simulink model "euler_equation_dave"  (R2021b)
settings: Solver=VariableStepAuto  StartTime=0.0  StopTime=30  MaxStep=0.01  RelTol=1e-3
values from neighbouring files (symbols this model uses):
  a = 2.4501e+4    (= 24501)    [heliocentric_plot.m]    (also in parameters_euler_equations_dave.m = 10500)
  e = 0.6665    [heliocentric_plot.m]    (also in parameters_euler_equations_dave.m = 0)
  Euler0131 = [0 pi/4 0]'    [parameters_euler_equations_dave.m]
  Euler0312 = [pi/4, 0, 0]'    [parameters_euler_equations_dave.m]
  h_versor = h ./ (h_norm)    [parameters_euler_equations_dave.m]
  I = [I_x_body, I_y_body, I_z_body]    [parameters_euler_equations_dave.m]
  i_0 = 0    [parameters_euler_equations_dave.m]
  J = diag (I)    [parameters_euler_equations_dave.m]
  J_inv = inv(J)    [parameters_euler_equations_dave.m]
  Mat_g = g .* S * 1e-09    [ghnorm.m]
  Mat_gsv = gsv .* S*  1e-09    [ghnorm.m]
  Mat_h = h .* S * 1e-09    [ghnorm.m]
  Mat_hsv = hsv .* S*  1e-09    [ghnorm.m]
  muP = astroConstants(13)    [parameters_euler_equations_dave.m]
  n = mat(:, 1)    [ghnorm.m]    (also in parameters_euler_equations_dave.m = 2*pi/T)
  N = max(mat (:, 2))    [ghnorm.m]    (also in parameters_euler_equations_dave.m = [n1 n2 n3 n4 n5 n6])
  n_sun = 2*pi/(365*24*3600)    (= 1.99238499086e-07)    [parameters_euler_equations_dave.m]    (also in srp.m = 1.99102127766e-07)
  R_sun = 149600000    [parameters_euler_equations_dave.m]
  Sat_dim = [a_body b_body c_body]    [parameters_euler_equations_dave.m]
  star1_in = [Sx(1); Sy(1); Sz(1)]    [parameters_euler_equations_dave.m]    (also in stars.m)
  star2_in = [Sx(2); Sy(2); Sz(2)]    [parameters_euler_equations_dave.m]    (also in stars.m)
  star3_in = [Sx(3); Sy(3); Sz(3)]    [parameters_euler_equations_dave.m]    (also in stars.m)
  theta_g0 = 0    [parameters_euler_equations_dave.m]
  true_anomaly0 = 0    [parameters_euler_equations_dave.m]
  Ts = 0.1    [parameters_euler_equations_dave.m]
  w0 = [wx, wy, wz]    [parameters_euler_equations_dave.m]
undefined symbols (not defined in the file or in its folder): A_SB, g_mat, h_mat, init_mjd2000, magnetic_torque, r0, t0, v0, vec_norm, we
libraries: sharedutil x13, vrlib x8, simulink_extras x6, sharedtransform x5, matrix_library x3, aerolibconvert2 x2, euler x1
(part 2 of 2)

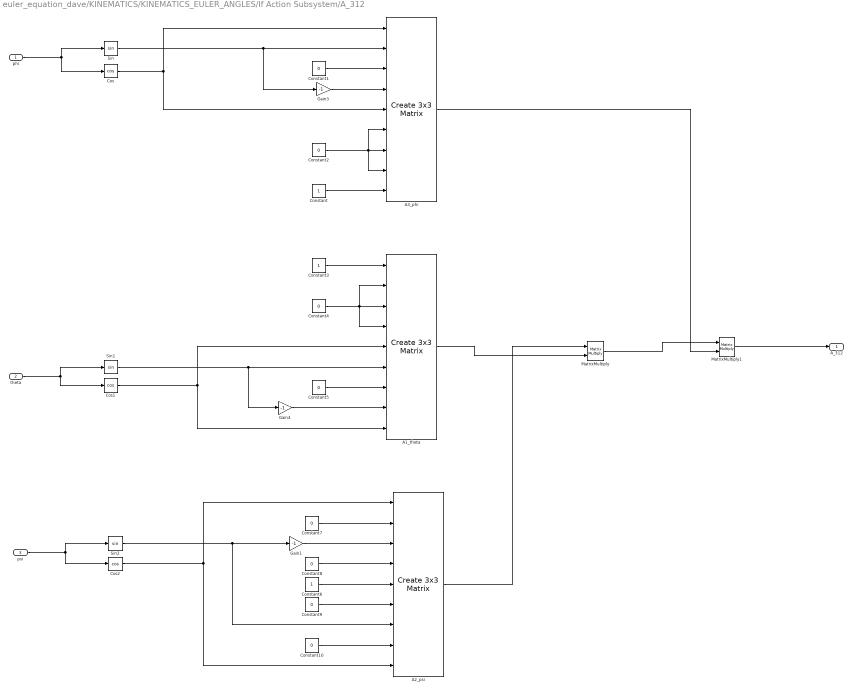
== system euler_equation_dave/KINEMATICS/KINEMATICS_EULER_ANGLES/If Action Subsystem/A_312 ==
  phi : Inport
  theta : Inport  Port=2
  psi : Inport  Port=3
  A1_theta : sharedutil/Create 3x3 Matrix  aMode=aMode
      settings: SourceProductBaseCode=AE,PW,DR,MT,UV,VE
  A2_psi : sharedutil/Create 3x3 Matrix  aMode=aMode
      settings: SourceProductBaseCode=AE,PW,DR,MT,UV,VE
  A3_phi : sharedutil/Create 3x3 Matrix  aMode=aMode
      settings: SourceProductBaseCode=AE,PW,DR,MT,UV,VE
  Constant : Constant
  Constant{1..2,4..5,7..10} (8 alike) : Constant  Value=0
  Constant3 : Constant
  Constant6 : Constant
  Cos : Trigonometry  Operator=cos
  Cos1 : Trigonometry  Operator=cos
  Cos2 : Trigonometry  Operator=cos
  Gain1 : Gain  Gain=-1
  Gain3 : Gain  Gain=-1
  Gain4 : Gain  Gain=-1
  MatrixMultiply : Product  Multiplication=Matrix(*)
  MatrixMultiply1 : Product  Multiplication=Matrix(*)
  Sin : Trigonometry
  Sin1 : Trigonometry
  Sin2 : Trigonometry
  A_312 : Outport
  wires:
  phi/1 -> Sin/1, Cos/1
  theta/1 -> Sin1/1, Cos1/1
  psi/1 -> Sin2/1, Cos2/1
  Cos/1 -> A3_phi/5, A3_phi/1
  Sin/1 -> A3_phi/2, Gain3/1
  Constant/1 -> A3_phi/9
  Constant1/1 -> A3_phi/3
  Constant2/1 -> A3_phi/8, A3_phi/6, A3_phi/7
  Constant3/1 -> A1_theta/1
  Constant4/1 -> A1_theta/4, A1_theta/3, A1_theta/2
  Cos1/1 -> A1_theta/5, A1_theta/9
  Constant5/1 -> A1_theta/7
  Cos2/1 -> A2_psi/9, A2_psi/1
  Constant7/1 -> A2_psi/2
  Constant9/1 -> A2_psi/6
  Constant8/1 -> A2_psi/4
  Constant6/1 -> A2_psi/5
  Sin2/1 -> A2_psi/7, Gain1/1
  Constant10/1 -> A2_psi/8
  A2_psi/1 -> MatrixMultiply/1
  A1_theta/1 -> MatrixMultiply/2
  MatrixMultiply/1 -> MatrixMultiply1/1
  A3_phi/1 -> MatrixMultiply1/2
  MatrixMultiply1/1 -> A_312/1
  Sin1/1 -> A1_theta/6, Gain4/1
  Gain3/1 -> A3_phi/4
  Gain4/1 -> A1_theta/8
  Gain1/1 -> A2_psi/3

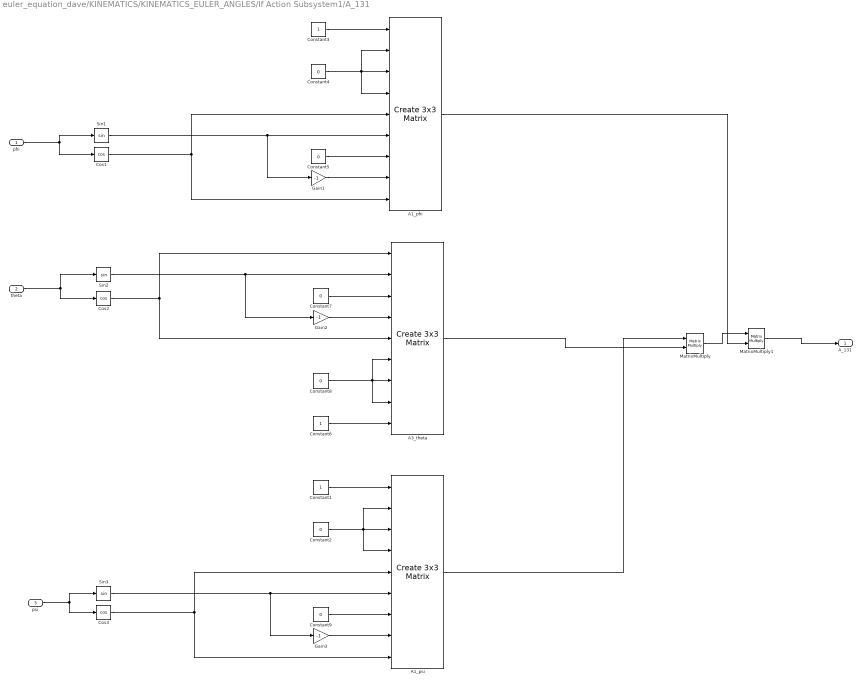
== system euler_equation_dave/KINEMATICS/KINEMATICS_EULER_ANGLES/If Action Subsystem1/A_131 ==
  phi : Inport
  theta : Inport  Port=2
  psi : Inport  Port=3
  A1_phi : sharedutil/Create 3x3 Matrix  aMode=aMode
      settings: SourceProductBaseCode=AE,PW,DR,MT,UV,VE
  A1_psi : sharedutil/Create 3x3 Matrix  aMode=aMode
      settings: SourceProductBaseCode=AE,PW,DR,MT,UV,VE
  A3_theta : sharedutil/Create 3x3 Matrix  aMode=aMode
      settings: SourceProductBaseCode=AE,PW,DR,MT,UV,VE
  Constant1 : Constant
  Constant{2,4..5,7..9} (6 alike) : Constant  Value=0
  Constant3 : Constant
  Constant6 : Constant
  Cos1 : Trigonometry  Operator=cos
  Cos2 : Trigonometry  Operator=cos
  Cos3 : Trigonometry  Operator=cos
  Gain1 : Gain  Gain=-1
  Gain2 : Gain  Gain=-1
  Gain3 : Gain  Gain=-1
  MatrixMultiply : Product  Multiplication=Matrix(*)
  MatrixMultiply1 : Product  Multiplication=Matrix(*)
  Sin1 : Trigonometry
  Sin2 : Trigonometry
  Sin3 : Trigonometry
  A_131 : Outport
  wires:
  Cos1/1 -> A1_phi/5, A1_phi/9
  Constant8/1 -> A3_theta/7, A3_theta/6, A3_theta/8
  Cos3/1 -> A1_psi/9, A1_psi/5
  Cos2/1 -> A3_theta/1, A3_theta/5
  Sin2/1 -> A3_theta/2, Gain2/1
  A3_theta/1 -> MatrixMultiply/2
  Gain1/1 -> A1_phi/8
  MatrixMultiply/1 -> MatrixMultiply1/1
  Constant9/1 -> A1_psi/7
  Sin1/1 -> Gain1/1, A1_phi/6
  Constant1/1 -> A1_psi/1
  Constant6/1 -> A3_theta/9
  Sin3/1 -> A1_psi/6, Gain3/1
  Gain3/1 -> A1_psi/8
  Gain2/1 -> A3_theta/4
  Constant4/1 -> A1_phi/4, A1_phi/3, A1_phi/2
  A1_phi/1 -> MatrixMultiply1/2
  Constant7/1 -> A3_theta/3
  A1_psi/1 -> MatrixMultiply/1
  Constant2/1 -> A1_psi/2, A1_psi/3, A1_psi/4
  Constant3/1 -> A1_phi/1
  Constant5/1 -> A1_phi/7
  MatrixMultiply1/1 -> A_131/1
  theta/1 -> Cos2/1, Sin2/1
  phi/1 -> Cos1/1, Sin1/1
  psi/1 -> Cos3/1, Sin3/1

== system euler_equation_dave/SENSORS/ATTITUDE DETERMINATION FOR GYROSCOPES/EULER ANGLES 131/PHI_DOT1 ==
  euler angles : Inport
  omega : Inport  Port=2
  Cos : Trigonometry  Operator=cos
  Cos1 : Trigonometry
  Demux : Demux  Outputs=3
  Demux1 : Demux  Outputs=3
  Divide : Product  Inputs=*/
  Product : Product
  Product1 : Product
  Sin : Trigonometry
  Sum : Sum  Inputs=-+
  Terminator : Terminator
  Terminator1 : Terminator
  phi_dot : Outport
  wires:
  omega/1 -> Demux/1
  euler angles/1 -> Demux1/1
  Demux1/2 -> Cos1/1
  Demux1/1 -> Terminator1/1
  Demux1/3 -> Cos/1, Sin/1
  Product/1 -> Sum/1
  Product1/1 -> Sum/2
  Sum/1 -> Divide/1
  Divide/1 -> phi_dot/1
  Demux/1 -> Terminator/1
  Cos1/1 -> Divide/2  "sin_theta!"
  Demux/3 -> Product1/2
  Sin/1 -> Product1/1
  Demux/2 -> Product/2  "w2"
  Cos/1 -> Product/1

== system euler_equation_dave/SENSORS/ATTITUDE DETERMINATION FOR GYROSCOPES/EULER ANGLES 131/PSI DOT1 ==
  Euler angles : Inport
  omega : Inport  Port=2
  Cos : Trigonometry  Operator=cos
  Cos1 : Trigonometry  Operator=cos
  Demux : Demux  Outputs=3
  Demux1 : Demux  Outputs=3
  Divide : Product  Inputs=*/
  Product : Product
  Product1 : Product
  Product2 : Product
  Sin : Trigonometry
  Sin1 : Trigonometry
  Sum : Sum  Inputs=+-
  Sum1 : Sum
  Terminator1 : Terminator
  psi_dot : Outport
  wires:
  Demux1/3 -> Cos/1, Sin/1
  Demux1/2 -> Sin1/1, Cos1/1
  Product/1 -> Sum/1
  Demux1/1 -> Terminator1/1
  Product1/1 -> Sum/2
  Euler angles/1 -> Demux1/1
  omega/1 -> Demux/1
  Divide/1 -> Sum1/1
  Sum1/1 -> psi_dot/1
  Sum/1 -> Product2/2  "w2*cos_psi-w3*sin_psi"
  Product2/1 -> Divide/1
  Demux/1 -> Sum1/2  "w1"
  Sin1/1 -> Divide/2  "sintheta!"
  Cos1/1 -> Product2/1  "cos_theta!"
  Demux/2 -> Product/1
  Cos/1 -> Product/2
  Demux/3 -> Product1/1
  Sin/1 -> Product1/2

== system euler_equation_dave/SENSORS/ATTITUDE DETERMINATION FOR GYROSCOPES/EULER ANGLES 131/THETA DOT1 ==
  euler angles : Inport
  omega : Inport  Port=2
  Cos : Trigonometry  Operator=cos
  Demux : Demux  Outputs=3
  Demux1 : Demux  Outputs=3
  Product : Product
  Product1 : Product
  Sin : Trigonometry
  Sum : Sum
  Terminator : Terminator
  Terminator1 : Terminator
  Terminator2 : Terminator
  theta_dot : Outport
  wires:
  Cos/1 -> Product/1
  Demux1/3 -> Sin/1, Cos/1
  Sin/1 -> Product1/2
  Product/1 -> Sum/1  "w3*cos_psi"
  Demux1/1 -> Terminator1/1
  omega/1 -> Demux/1
  Sum/1 -> theta_dot/1
  euler angles/1 -> Demux1/1
  Product1/1 -> Sum/2  "w2*sin_psi"
  Demux1/2 -> Terminator2/1
  Demux/1 -> Terminator/1
  Demux/3 -> Product/2
  Demux/2 -> Product1/1  "w2"

== system euler_equation_dave/SENSORS/ATTITUDE DETERMINATION FOR GYROSCOPES/EULER ANGLES 312/PHI_DOT ==
  euler angles : Inport
  omega : Inport  Port=2
  Cos : Trigonometry  Operator=cos
  Cos1 : Trigonometry  Operator=cos
  Demux : Demux  Outputs=3
  Demux1 : Demux  Outputs=3
  Divide : Product  Inputs=*/
  Product : Product
  Product1 : Product
  Sin : Trigonometry
  Sum : Sum  Inputs=+-
  Terminator : Terminator
  Terminator1 : Terminator
  phi_dot : Outport
  wires:
  omega/1 -> Demux/1
  Demux/2 -> Terminator/1  "w2"
  Demux/1 -> Product1/1
  euler angles/1 -> Demux1/1
  Demux1/2 -> Cos1/1
  Demux1/1 -> Terminator1/1
  Demux1/3 -> Cos/1, Sin/1
  Sin/1 -> Product1/2
  Cos/1 -> Product/1
  Demux/3 -> Product/2
  Product/1 -> Sum/1
  Cos1/1 -> Divide/2  "cos_theta!"
  Product1/1 -> Sum/2
  Sum/1 -> Divide/1
  Divide/1 -> phi_dot/1

== system euler_equation_dave/SENSORS/ATTITUDE DETERMINATION FOR GYROSCOPES/EULER ANGLES 312/PSI DOT ==
  Euler angles : Inport
  omega : Inport  Port=2
  Cos : Trigonometry  Operator=cos
  Cos1 : Trigonometry  Operator=cos
  Demux : Demux  Outputs=3
  Demux1 : Demux  Outputs=3
  Divide : Product  Inputs=*/
  Product : Product
  Product1 : Product
  Product2 : Product
  Sin : Trigonometry
  Sin1 : Trigonometry
  Sum : Sum  Inputs=+-
  Sum1 : Sum  Inputs=-+
  Terminator1 : Terminator
  psi_dot : Outport
  wires:
  Demux1/3 -> Cos/1, Sin/1
  Demux1/2 -> Sin1/1, Cos1/1
  Product/1 -> Sum/1
  Demux1/1 -> Terminator1/1
  Cos1/1 -> Divide/2  "cos_theta!"
  Product1/1 -> Sum/2
  Euler angles/1 -> Demux1/1
  omega/1 -> Demux/1
  Demux/2 -> Sum1/2  "w2"
  Divide/1 -> Sum1/1
  Sum1/1 -> psi_dot/1
  Demux/3 -> Product/2
  Cos/1 -> Product/1
  Demux/1 -> Product1/1
  Sin/1 -> Product1/2
  Sin1/1 -> Product2/1
  Sum/1 -> Product2/2  "w3*cos_psi-w1*sin_psi"
  Product2/1 -> Divide/1

== system euler_equation_dave/SENSORS/ATTITUDE DETERMINATION FOR GYROSCOPES/EULER ANGLES 312/THETA DOT ==
  euler angles : Inport
  omega : Inport  Port=2
  Cos : Trigonometry  Operator=cos
  Demux : Demux  Outputs=3
  Demux1 : Demux  Outputs=3
  Product : Product
  Product1 : Product
  Sin : Trigonometry
  Sum : Sum
  Terminator : Terminator
  Terminator1 : Terminator
  Terminator2 : Terminator
  theta_dot : Outport
  wires:
  Cos/1 -> Product/1
  Demux/2 -> Terminator/1  "w2"
  Demux1/3 -> Sin/1, Cos/1
  Sin/1 -> Product1/2
  Product/1 -> Sum/1  "w1*cos_psi"
  Demux1/1 -> Terminator1/1
  omega/1 -> Demux/1
  Sum/1 -> theta_dot/1
  euler angles/1 -> Demux1/1
  Product1/1 -> Sum/2  "w3*sin_psi"
  Demux1/2 -> Terminator2/1
  Demux/1 -> Product/2
  Demux/3 -> Product1/1

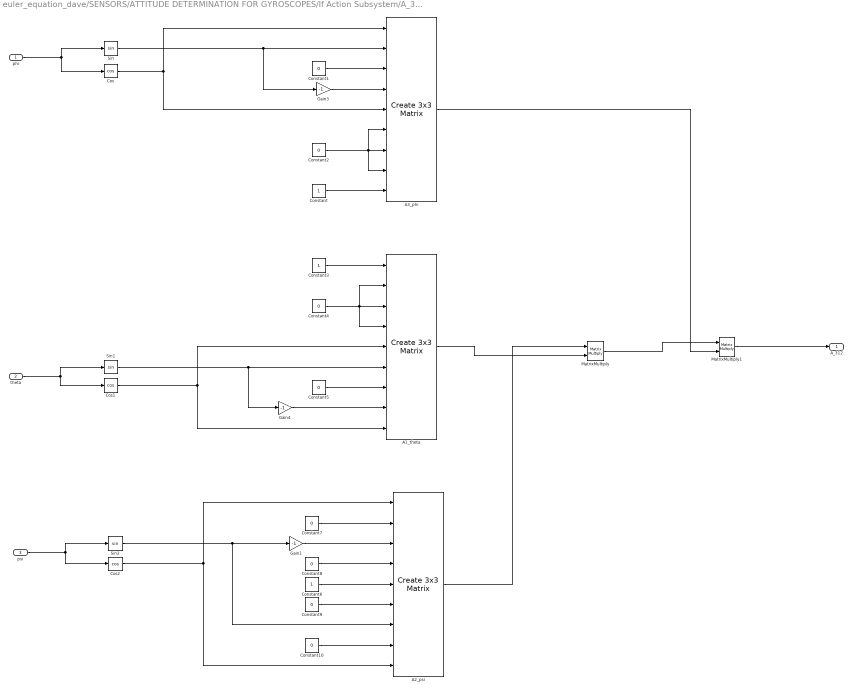
== system euler_equation_dave/SENSORS/ATTITUDE DETERMINATION FOR GYROSCOPES/If Action Subsystem/A_312 ==
  phi : Inport
  theta : Inport  Port=2
  psi : Inport  Port=3
  A1_theta : sharedutil/Create 3x3 Matrix  aMode=aMode
      settings: SourceProductBaseCode=AE,PW,DR,MT,UV,VE
  A2_psi : sharedutil/Create 3x3 Matrix  aMode=aMode
      settings: SourceProductBaseCode=AE,PW,DR,MT,UV,VE
  A3_phi : sharedutil/Create 3x3 Matrix  aMode=aMode
      settings: SourceProductBaseCode=AE,PW,DR,MT,UV,VE
  Constant : Constant
  Constant{1..2,4..5,7..10} (8 alike) : Constant  Value=0
  Constant3 : Constant
  Constant6 : Constant
  Cos : Trigonometry  Operator=cos
  Cos1 : Trigonometry  Operator=cos
  Cos2 : Trigonometry  Operator=cos
  Gain1 : Gain  Gain=-1
  Gain3 : Gain  Gain=-1
  Gain4 : Gain  Gain=-1
  MatrixMultiply : Product  Multiplication=Matrix(*)
  MatrixMultiply1 : Product  Multiplication=Matrix(*)
  Sin : Trigonometry
  Sin1 : Trigonometry
  Sin2 : Trigonometry
  A_312 : Outport
  wires:
  phi/1 -> Sin/1, Cos/1
  theta/1 -> Sin1/1, Cos1/1
  psi/1 -> Sin2/1, Cos2/1
  Cos/1 -> A3_phi/5, A3_phi/1
  Sin/1 -> A3_phi/2, Gain3/1
  Constant/1 -> A3_phi/9
  Constant1/1 -> A3_phi/3
  Constant2/1 -> A3_phi/8, A3_phi/6, A3_phi/7
  Constant3/1 -> A1_theta/1
  Constant4/1 -> A1_theta/4, A1_theta/3, A1_theta/2
  Cos1/1 -> A1_theta/5, A1_theta/9
  Constant5/1 -> A1_theta/7
  Cos2/1 -> A2_psi/9, A2_psi/1
  Constant7/1 -> A2_psi/2
  Constant9/1 -> A2_psi/6
  Constant8/1 -> A2_psi/4
  Constant6/1 -> A2_psi/5
  Sin2/1 -> A2_psi/7, Gain1/1
  Constant10/1 -> A2_psi/8
  A2_psi/1 -> MatrixMultiply/1
  A1_theta/1 -> MatrixMultiply/2
  MatrixMultiply/1 -> MatrixMultiply1/1
  A3_phi/1 -> MatrixMultiply1/2
  MatrixMultiply1/1 -> A_312/1
  Sin1/1 -> A1_theta/6, Gain4/1
  Gain3/1 -> A3_phi/4
  Gain4/1 -> A1_theta/8
  Gain1/1 -> A2_psi/3

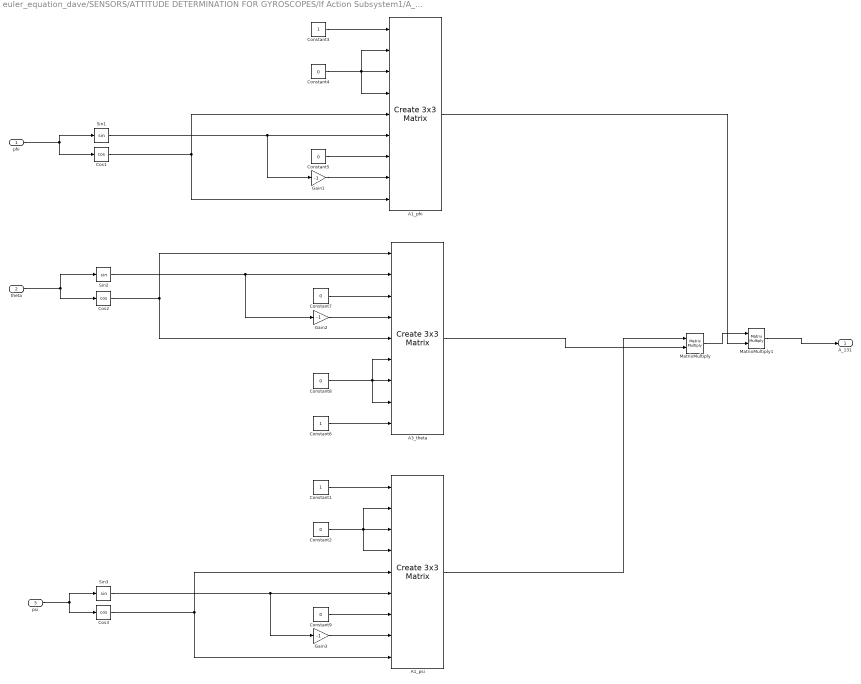
== system euler_equation_dave/SENSORS/ATTITUDE DETERMINATION FOR GYROSCOPES/If Action Subsystem1/A_131 ==
  phi : Inport
  theta : Inport  Port=2
  psi : Inport  Port=3
  A1_phi : sharedutil/Create 3x3 Matrix  aMode=aMode
      settings: SourceProductBaseCode=AE,PW,DR,MT,UV,VE
  A1_psi : sharedutil/Create 3x3 Matrix  aMode=aMode
      settings: SourceProductBaseCode=AE,PW,DR,MT,UV,VE
  A3_theta : sharedutil/Create 3x3 Matrix  aMode=aMode
      settings: SourceProductBaseCode=AE,PW,DR,MT,UV,VE
  Constant1 : Constant
  Constant{2,4..5,7..9} (6 alike) : Constant  Value=0
  Constant3 : Constant
  Constant6 : Constant
  Cos1 : Trigonometry  Operator=cos
  Cos2 : Trigonometry  Operator=cos
  Cos3 : Trigonometry  Operator=cos
  Gain1 : Gain  Gain=-1
  Gain2 : Gain  Gain=-1
  Gain3 : Gain  Gain=-1
  MatrixMultiply : Product  Multiplication=Matrix(*)
  MatrixMultiply1 : Product  Multiplication=Matrix(*)
  Sin1 : Trigonometry
  Sin2 : Trigonometry
  Sin3 : Trigonometry
  A_131 : Outport
  wires:
  Cos1/1 -> A1_phi/5, A1_phi/9
  Constant8/1 -> A3_theta/7, A3_theta/6, A3_theta/8
  Cos3/1 -> A1_psi/9, A1_psi/5
  Cos2/1 -> A3_theta/1, A3_theta/5
  Sin2/1 -> A3_theta/2, Gain2/1
  A3_theta/1 -> MatrixMultiply/2
  Gain1/1 -> A1_phi/8
  MatrixMultiply/1 -> MatrixMultiply1/1
  Constant9/1 -> A1_psi/7
  Sin1/1 -> Gain1/1, A1_phi/6
  Constant1/1 -> A1_psi/1
  Constant6/1 -> A3_theta/9
  Sin3/1 -> A1_psi/6, Gain3/1
  Gain3/1 -> A1_psi/8
  Gain2/1 -> A3_theta/4
  Constant4/1 -> A1_phi/4, A1_phi/3, A1_phi/2
  A1_phi/1 -> MatrixMultiply1/2
  Constant7/1 -> A3_theta/3
  A1_psi/1 -> MatrixMultiply/1
  Constant2/1 -> A1_psi/2, A1_psi/3, A1_psi/4
  Constant3/1 -> A1_phi/1
  Constant5/1 -> A1_phi/7
  MatrixMultiply1/1 -> A_131/1
  theta/1 -> Cos2/1, Sin2/1
  phi/1 -> Cos1/1, Sin1/1
  psi/1 -> Cos3/1, Sin3/1

== system euler_equation_dave/ENVIRONMENT/MAGNETIC TORQUE/magnetic_torque/r_N_to_lat_lon_lst/latitude ==
  r : Inport
  z : Inport  Port=2
  Asin : Trigonometry  Operator=asin
  Divide : Product  Inputs=*/
  Radians to Degrees : simulink_extras/Transformations/Radians to Degrees
  lat : Outport
  wires:
  Radians to Degrees/1 -> lat/1  "lat"
  Asin/1 -> Radians to Degrees/1  "lat"
  r/1 -> Divide/2
  Divide/1 -> Asin/1  "z/r"
  z/1 -> Divide/1

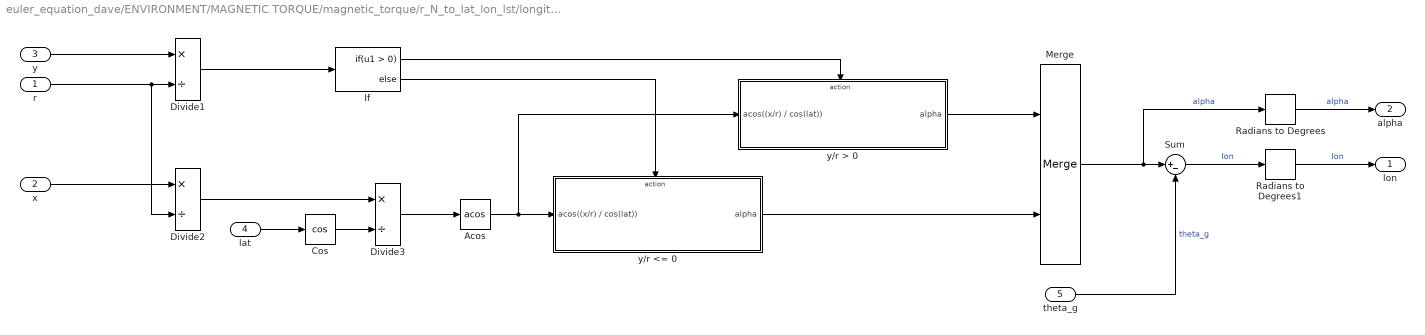
== system euler_equation_dave/ENVIRONMENT/MAGNETIC TORQUE/magnetic_torque/r_N_to_lat_lon_lst/longitude_LST ==
  r : Inport
  x : Inport  Port=2
  y : Inport  Port=3
  lat : Inport  Port=4
  theta_g : Inport  Port=5
  Acos : Trigonometry  Operator=acos
  Cos : Trigonometry  Operator=cos
  Divide1 : Product  Inputs=*/
  Divide2 : Product  Inputs=*/
  Divide3 : Product  Inputs=*/
  If : If
  Merge : Merge
  Radians to Degrees : simulink_extras/Transformations/Radians to Degrees
  Radians to Degrees1 : simulink_extras/Transformations/Radians to Degrees
  Sum : Sum  Inputs=|+-
  y/r <= 0 : Subsystem  TreatAsAtomicUnit=on
  "y/r > 0 " : Subsystem  TreatAsAtomicUnit=on
  lon : Outport
  alpha : Outport  Port=2
  wires:
  Radians to Degrees1/1 -> lon/1  "lon"
  Radians to Degrees/1 -> alpha/1  "alpha"
  Acos/1 -> "y/r > 0 "/1(acos((x/r) / cos(lat))), y/r <= 0/1(acos((x/r) / cos(lat)))
  lat/1 -> Cos/1
  Cos/1 -> Divide3/2
  Divide3/1 -> Acos/1
  Divide2/1 -> Divide3/1
  x/1 -> Divide2/1
  Sum/1 -> Radians to Degrees1/1  "lon"
  theta_g/1 -> Sum/2  "theta_g"
  Merge/1 -> Sum/1, Radians to Degrees/1  "alpha"
  y/r <= 0/1(alpha) -> Merge/2
  "y/r > 0 "/1(alpha) -> Merge/1
  If/2 -> y/r <= 0/Action
  If/1 -> "y/r > 0 "/Action
  y/1 -> Divide1/1
  r/1 -> Divide2/2, Divide1/2
  Divide1/1 -> If/1

== system euler_equation_dave/ENVIRONMENT/MAGNETIC TORQUE/magnetic_torque/r_N_to_lat_lon_lst/r_norm ==
  vector : Inport
  Dot Product : DotProduct  InputSameDT=on  OutDataTypeStr=Inherit: Inherit via internal rule
  Square Root : Sqrt  SaturateOnIntegerOverflow=on
  norm : Outport
  wires:
  Dot Product/1 -> Square Root/1
  vector/1 -> Dot Product/2, Dot Product/1
  Square Root/1 -> norm/1

== system euler_equation_dave/ENVIRONMENT/MAGNETIC TORQUE/magnetic_torque/r_N_to_lat_lon_lst/longitude_LST/y//r <= 0 ==
  acos((x/r) / cos(lat)) : Inport
  Action Port : ActionPort  ActionPortLabel=else
  2*pi : Constant  Value=2*pi
  Sum : Sum  Inputs=|-+
  alpha : Outport
  wires:
  Sum/1 -> alpha/1
  2*pi/1 -> Sum/2
  acos((x/r) / cos(lat))/1 -> Sum/1

== system euler_equation_dave/ENVIRONMENT/MAGNETIC TORQUE/magnetic_torque/r_N_to_lat_lon_lst/longitude_LST/y//r > 0  ==
  acos((x/r) / cos(lat)) : Inport
  Action Port : ActionPort  ActionPortLabel=if(u1 > 0)
  alpha : Outport
  wires:
  acos((x/r) / cos(lat))/1 -> alpha/1

== matlab function euler_equation_dave/ENVIRONMENT/SRP/MATLAB Function ==
  data: Sat_dim input; M output; N input; A_BN input; t input


 % SOLAR RADIATION PRESSURE TORQUE CALCULATION
%
% computes the solar radiation pressure torque applied on a cubic
% spacecraft based on its dimension, orientation, and time of the
% year to compute solar position

% /!\ this is only the first version, aka experimental draft
% TO-DO : We should account for the planet shadowing on the spacecraft for
% the next version, as this model only represents the sun and the satellite
% in the system.
% SOLAR RADIATION PRESSURE TORQUE CALCULATION
%
% computes the solar radiation pressure torque applied on a cubic
% spacecraft based on its dimension, orientation, and time of the
% year to compute solar position

% /!\ this is only the first version, aka experimental draft
% TO-DO : We should account for the planet shadowing on the spacecraft for
% the next version, as this model only represents the sun and the satellite
% in the system.

function M= srp(Sat_dim,N,A_BN,t)
    % Sat_dim is the cubic satellite dimentions [x y z]' in m
    % N is the set of faces' orientations (normals) of the satellite
    % given as [n1 n2 n3 n4 n5 n6] with ni = [xi yi zi]'
    % A_BN is the rotation matrix between the satellite and the inertial frame
    % t is the time of the year in s
    
    % reflection coefficients definition
    rho_s = 0.5; % [no unit] specular refelection coefficient
    rho_d = 0.1; % [no unit] diffuse refelection coefficient

    %faces surface definition
    surface = [Sat_dim(2)*Sat_dim(3), Sat_dim(1)*Sat_dim(3), Sat_dim(1)*Sat_dim(2)];
    
    %pressure definition
    c = 299792458; % [m/s] light speed
    Fe = 1358; % [W/m2] power per unit surface
    P = Fe/c; % [Pa] Solar Radiation Pressure
    
    %sun orientation definition
    T = 365.25*24*3600; % [s] one year's time span
    n_sun = 2*pi/T; % [rad/s] sun's rotation period around earth
    Rs = 150e9; % [m] earth/sun distance
    epsilon = 23.45*pi/180; % [rad]
    S_B = A_BN*[cos(n_sun*t) , sin(n_sun*t)*cos(epsilon) , sin(n_sun*t)*sin(epsilon)]';
    
    %computation
    M = zeros(3,1); % SRP-induced torque
    for n=1:6

        if dot(S_B, N(:, n)) > 0
            A = surface(mod(n-1,3)+1);
            F = -P*A*dot(S_B,N(:,n))*((1-rho_s)*S_B+(2*rho_s*dot(S_B,N(:,n))+(2/3)*rho_d)*N(:,n));
            M = M + cross((Sat_dim(mod(n-1,3)+1)/2)*N(:,n),F);
        else
            M = M + zeros(3,1);
        end
        
    end
end

== matlab function euler_equation_dave/ENVIRONMENT/MAGNETIC TORQUE/Subsystem/MATLAB Function ==
  data: r_N input; theta_g0 input; t input; lat output; long output; days_mission output
function [lat, long, days_mission] = gdt(r_N, theta_g0, t)




% define x, y, z position in inertial reference frame and Earth rotation
% speed
we = deg2rad(15.04 / 3600);

% day0 = 0; %time of departure of mission from Jan, 01 2020 
% secondsinday = 24*3600;
% days_mission = (t/secondsinday + day0);


x= r_N(1);
y = r_N(2);
z = r_N(3);
r_norm  = norm (r_N);

% declination
delta = asin (z ./ r_norm);

% right ascension
alfa = acos ((x./r_norm)./(cos(delta))) .* sign (y./r_norm) + 2*pi*(y./r_norm < 0);

%define theta Greenwich

t0 = 0; 
theta_g = theta_g0 + we * (t - t0); % theta_g at t time of simulation generates a long and lat corresponding to t time of simulation

% longitude
long  = mod(alfa - theta_g, 2*pi); %respects  both orbital mechanics and code for magnetic field notation: positive east from greenwich meridian

%latitude
lat = mod(delta, 2*pi); %respects both orbital mechanics and code for magnetic field notation: positive north from equator



end

== matlab function euler_equation_dave/ENVIRONMENT/MAGNETIC TORQUE/Subsystem/MATLAB Function1 ==
  data: Mat_h input; Mat_g input; Mat_gsv input; Mat_hsv input; r_N input; Br output; lat input; long input; days_mission input; Bt output; Bp output
function [Br, Bt, Bp] = magnet(Mat_h, Mat_g, Mat_gsv, Mat_hsv, r_N, lat, long, days_mission)

    
% Inputs
%lots of IGRF coefficients+secular variations
% r_N distance from Earth center in inertial reference frame
% lat: Latitude measured in degrees positive from equator
% long: Longitude measured in degrees positive east from Greenwich
% days_mission: Decimal days since January 1, 2000
%
% Outputs - magnetic field strength in local tangential coordinates
% Br B in radial direction
% Bt B in theta direction
% Bp B in phi direction
% Checks to see if located at either pole to avoid singularities
if (lat>deg2rad(-0.00000001) && lat<deg2rad(0.00000001))
lat=deg2rad(0.00000001);
elseif(lat<deg2rad(180.00000001) && lat>deg2rad(179.99999999))
lat=deg2rad(179.99999999);
end

% % The angles must be converted from degrees into radians
lat=(90-rad2deg(lat))*pi/180;
% long = long*pi/180;

a=6371.2; % Reference radius used in IGRF

% This section of the code simply reads in the g and h Schmidt
% quasi-normalized coefficients
% [gn, gm, gvali, gsvi] = textread(’igrfSg.txt’,’%f %f %f %f’);
% [hn, hm, hvali, hsvi] = textread(’igrfSh.txt’,’%f %f %f %f’);


N=min(size(Mat_g));
g=zeros(N,N+1);
h=zeros(N,N+1);
g = Mat_g Mat_gsv*days_mission/365;
h = Mat_h Mat_hsv*days_mission/365;
%since I saved both the results of g and h coefficients and secular
%variations for g and h in matrices, I can just sum them

% for x=1:length(Mat_g)
% g(Mat_g(x),Mat_g(x)+1) = Mat_g(x) + Mat_gsv(x)*days/365;
% h(Mat_h(x),Mat_h(x)+1) = Mat_h(x) + Mat_hsv(x)*days/365;
% end



% Initialize each of the variables
% Br B in the radial driection
% Bt B in the theta direction
% Bp B in the phi direction


% P The associated Legendre polynomial evaluated at cos(theta)
% The nomenclature for the recursive values generally follows
% the form P10 = P(n-1,m-0)
% dP The partial derivative of P with respect to theta
Br=0; Bt=0; Bp=0;
P11=1; P10=P11;
dP11=0; dP10=dP11;


%since the matrices have length 14, but indexes n and m go up to 13 only.
for m=0:N
for n=1:N
if m<=n
% Calculate Legendre polynomials and derivatives recursively
if n==m
P2 = sin(lat)*P11;
dP2 = sin(lat)*dP11 + cos(lat)*P11;
P11=P2; P10=P11; P20=0;
dP11=dP2; dP10=dP11; dP20=0;
elseif n==1
P2 = cos(lat)*P10;
dP2 = cos(lat)*dP10 - sin(lat)*P10;
P20=P10; P10=P2;
dP20=dP10; dP10=dP2;
else
K = ((n-1)^2-m^2)/((2*n-1)*(2*n-3));
P2 = cos(lat)*P10 - K*P20;
dP2 = cos(lat)*dP10 - sin(lat)*P10 - K*dP20;
P20=P10; P10=P2;
dP20=dP10; dP10=dP2;
end


% Calculate Br, Bt, and Bp
Br = Br + (a/r_N)^(n+2)*(n+1)*((g(n,m+1)*cos(m*long) + h(n,m+1)*sin(m*long))*P2);
Bt = Bt + (a/r_N)^(n+2)*((g(n,m+1)*cos(m*long) + h(n,m+1)*sin(m*long))*dP2);
Bp = Bp + (a/r_N)^(n+2)*(m*(-g(n,m+1)*sin(m*long) + h(n,m+1)*cos(m*long))* P2);

end
end
end
[Br,Bt,Bp] = [Br;-Bt;-Bp/sin(lat)];

end

== matlab function euler_equation_dave/ENVIRONMENT/MAGNETIC TORQUE/Subsystem/MATLAB Function2 ==
  data: Br input; Bx output; Bt input; Bp input; LST input; lat input; By output; Bz output



function [Bx,By,Bz] = msph2inert(Br,Bt,Bp,LST,lat)
% Inputs
% Br B in radial direction | Magnetic field strength (B)
% Bt B in theta direction | in local tangential coordinates
% Bp B in phi direction |
% LST Local sidereal time of location (in degrees)
% lat Latitude measured positive north from equator (in degrees)
% Outputs
% Bx B in x-direction | Magnetic field strength (B)
% By B in y-direction | in geocentric inertial coordinates
% Bz B in z-direction |
% Angle conversion to radians
% lat=lat*pi/180; LST=LST*pi/180;
% Coordinate transformation
Bx = (Br*cos(lat)+Bt*sin(lat))*cos(LST) - Bp*sin(LST);
By = (Br*cos(lat)+Bt*sin(lat))*sin(LST) + Bp*cos(LST);
Bz = (Br*sin(lat)+Bt*cos(lat));

end

== matlab function euler_equation_dave/ENVIRONMENT/MAGNETIC TORQUE/magnetic_torque/MATLAB Function ==
  data: r input; B output; lat input; lon input; alpha input; mjd2000 input; g_mat input; h_mat input
function B = magnet(r, lat, lon, alpha, mjd2000, g_mat, h_mat)
    % Inputs
    % r Geocentric radius
    % lat Latitude measured in degrees positive from equator
    % lon Longitude measured in degrees positive east from Greenwich
    % alpha Local sidereal time of location (in degrees)
    % mjd2000 Decimal days since January 1, 2000
    %
    % Outputs
    % Bx B in x-direction | Magnetic field strength (B)
    % By B in y-direction | in geocentric inertial coordinates
    % Bz B in z-direction |

    % Checks to see if located at either pole to avoid singularities
    if (lat > -0.00000001 && lat < 0.00000001)
        lat = 0.00000001;
    elseif(lat < 180.00000001 && lat > 179.99999999)
        lat = 179.99999999;
    end

    % The angles must be converted from degrees into radians
    co_lat = (90 - lat) * pi/180;  % co-latitude
    lon = lon * pi/180;
    a = 6371.2; % Reference radius used in IGRF

    % This section of the code simply reads in the g and h Schmidt
    % quasi-normalized coefficients
    gn = g_mat(:, 1); gm = g_mat(:, 2); gvali = g_mat(:, 3); gsvi = g_mat(:, 4);
    hn = h_mat(:, 1); hm = h_mat(:, 2); hvali = h_mat(:, 3); hsvi = h_mat(:, 4);

    N = max(gn);
    g = zeros(N, N+1);
    h = zeros(N, N+1);

    for x=1:length(gn)
        g(gn(x), gm(x)+1) = gvali(x) + gsvi(x) * mjd2000/365;
        h(hn(x), hm(x)+1) = hvali(x) + hsvi(x) * mjd2000/365;
    end

    % Initialize each of the variables
    % Br B in the radial driection
    % Bt B in the theta direction
    % Bp B in the phi direction
    % P The associated Legendre polynomial evaluated at cos(theta)
    % The nomenclature for the recursive values generally follows
    % the form P10 = P(n-1,m-0)
    % dP The partial derivative of P with respect to theta
    Br = 0; Bt = 0; Bp = 0;
    P11 = 1; P10 = P11; P20 = P10;
    dP11 = 0; dP10 = dP11; dP20 = dP10;

    for m = 0:N
        for n = 1:N
            if m <= n
                % Calculate Legendre polynomials and derivatives recursively
                if n == m
                    P2 = sin(co_lat)*P11;
                    dP2 = sin(co_lat)*dP11 + cos(co_lat)*P11;
                    P11 = P2; P10 = P11; P20 = 0;
                    dP11 = dP2; dP10 = dP11; dP20 = 0;
                elseif n == 1
                    P2 = cos(co_lat)*P10;
                    dP2 = cos(co_lat)*dP10 - sin(co_lat)*P10;
                    P20 = P10; P10 = P2;
                    dP20 = dP10; dP10 = dP2;
                else
                    K = ((n-1)^2-m^2) / ((2*n-1)*(2*n-3));
                    P2 = cos(co_lat)*P10 - K*P20;
                    dP2 = cos(co_lat)*dP10 - sin(co_lat)*P10 - K*dP20;
                    P20 = P10; P10 = P2;
                    dP20 = dP10; dP10 = dP2;
                end

                % Calculate Br, Bt, and Bp
                Br = Br + (a/r)^(n+2)*(n+1)*...
                ((g(n,m+1)*cos(m*lon) + h(n,m+1)*sin(m*lon))*P2);

                Bt = Bt + (a/r)^(n+2)*...
                ((g(n,m+1)*cos(m*lon) + h(n,m+1)*sin(m*lon))*dP2);

                Bp = Bp + (a/r)^(n+2)*...
                (m*(-g(n,m+1)*sin(m*lon) + h(n,m+1)*cos(m*lon))* P2);
            end
        end
    end
    Bt = -Bt; Bp = -Bp/sin(co_lat);

    % Angle conversion to radians
    lat = lat * pi/180; alpha = alpha * pi/180;
    % Coordinate transformation
    Bx = (Br*cos(lat)+Bt*sin(lat))*cos(alpha) - Bp*sin(alpha);
    By = (Br*cos(lat)+Bt*sin(lat))*sin(alpha) + Bp*cos(alpha);
    Bz = (Br*sin(lat)+Bt*cos(lat));

    B = [Bx; By; Bz];
end
